simulink model "Boost_Converter_e"  (R2018b)
settings: Solver=VariableStepAuto  StartTime=0.0  StopTime=0.05  RelTol=1e-3
libraries: powerlib x21, pePowerMeasurement x4, powerlib_meascontrol x2
settings Model: Creator=Asus  LastModifiedBy=Asus

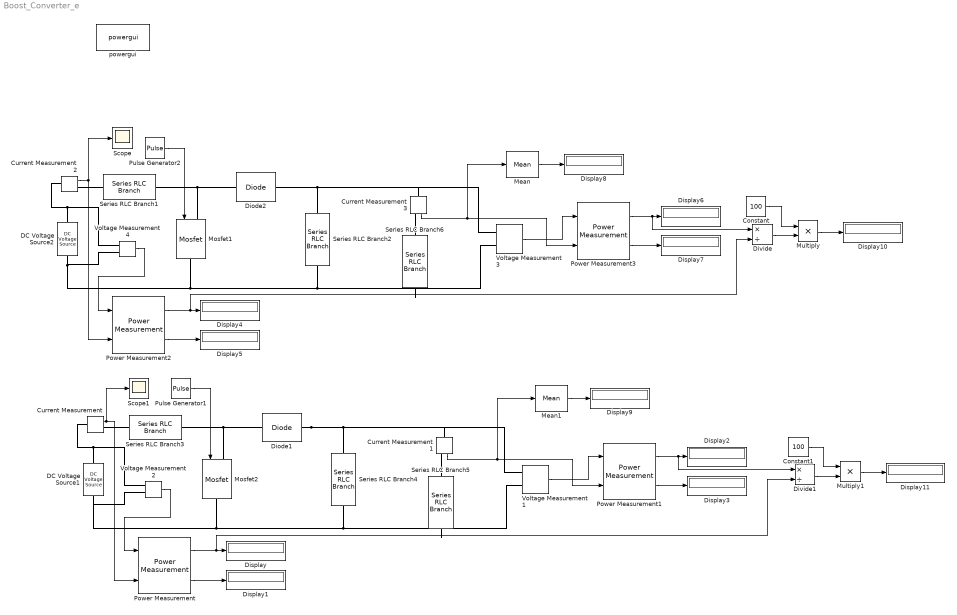
== system Boost_Converter_e ==
  Constant : Constant  Value=100
  Constant1 : Constant  Value=100
  Current Measurement{,1..3} (4 alike) : powerlib/Measurements/Current Measurement  PhasorSimulation=off  OutputType=Complex  PSBequivalent=0
  DC Voltage Source1 : powerlib/Electrical Sources/DC Voltage Source  Amplitude=15  Measurements=None
  DC Voltage Source2 : powerlib/Electrical Sources/DC Voltage Source  Amplitude=15  Measurements=None
  Diode1 : powerlib/Power Electronics/Diode  Ron=0  Lon=0  Vf=0  IC=0  UseSnubber=0  Rs=inf  Cs=inf  Measurements=off
  Diode2 : powerlib/Power Electronics/Diode  Ron=0  Lon=0  Vf=0  IC=0  UseSnubber=0  Rs=inf  Cs=inf  Measurements=off
  Display{,1..11} (12 alike) : Display
  Divide : Product  Inputs=*/
  Divide1 : Product  Inputs=*/
  Mean : powerlib_meascontrol/Measurements/Mean  Freq=500000  Vinit=0  Ts=0
  Mean1 : powerlib_meascontrol/Measurements/Mean  Freq=500000  Vinit=0  Ts=0
  Mosfet1 : powerlib/Power Electronics/Mosfet  Ron=0  Lon=0  Rd=0  Vfd=0  IC=0  Rs=inf  Cs=inf  Measurements=off
  Mosfet2 : powerlib/Power Electronics/Mosfet  Ron=0  Lon=0  Rd=0  Vfd=0  IC=0  Rs=inf  Cs=inf  Measurements=off
  Multiply : Product
  Multiply1 : Product
  Power Measurement{,1..3} (4 alike) : pePowerMeasurement/Power Measurement  LabelModeActiveChoice=Continuous  F=50000  K=[0 1 2 3]  Ts=0
  Pulse Generator1 : DiscretePulseGenerator  PulseType=Time based  Period=1/500000  PulseWidth=37.5
  Pulse Generator2 : DiscretePulseGenerator  PulseType=Time based  Period=1/500000  PulseWidth=37.5
  Scope : Scope
  Scope1 : Scope
  Series RLC Branch1 : powerlib/Elements/Series RLC Branch  LConnTagsString=__new0  RConnTagsString=__new0  BranchType=L  Resistance=57e-3  Inductance=8.53e-6  SetiL0=off  InitialCurrent=0  Capacitance=1e-6  Setx0=off  InitialVoltage=0  Measurements=None
  Series RLC Branch2 : powerlib/Elements/Series RLC Branch  LConnTagsString=__new0  RConnTagsString=__new0  BranchType=C  Resistance=1  Inductance=1e-3  SetiL0=off  InitialCurrent=0  Capacitance=3.125e-6  Setx0=off  InitialVoltage=0  Measurements=None
  Series RLC Branch3 : powerlib/Elements/Series RLC Branch  LConnTagsString=__new0  RConnTagsString=__new0  BranchType=RL  Resistance=57e-3  Inductance=8.53e-6  SetiL0=off  InitialCurrent=0  Capacitance=1e-6  Setx0=off  InitialVoltage=0  Measurements=None
  Series RLC Branch4 : powerlib/Elements/Series RLC Branch  LConnTagsString=__new0  RConnTagsString=__new0  BranchType=C  Resistance=1  Inductance=1e-3  SetiL0=off  InitialCurrent=0  Capacitance=3.125e-6  Setx0=off  InitialVoltage=0  Measurements=None
  Series RLC Branch5 : powerlib/Elements/Series RLC Branch  LConnTagsString=__new0  RConnTagsString=__new0  BranchType=R  Resistance=12  Inductance=1e-3  SetiL0=off  InitialCurrent=0  Capacitance=1e-6  Setx0=off  InitialVoltage=0  Measurements=None
  Series RLC Branch6 : powerlib/Elements/Series RLC Branch  LConnTagsString=__new0  RConnTagsString=__new0  BranchType=R  Resistance=12  Inductance=1e-3  SetiL0=off  InitialCurrent=0  Capacitance=1e-6  Setx0=off  InitialVoltage=0  Measurements=None
  Voltage Measurement{1..4} (4 alike) : powerlib/Measurements/Voltage Measurement  PhasorSimulation=off  OutputType=Complex  PSBequivalent=0
  powergui : powerlib/powergui  Priority=1  SimulationMode=Continuous  SampleTime=50e-6  frequency=60  Iterations=50  frequencyindice=0  Pbase=100e6  ErrMax=1e-4  UnitsV=kV  UnitsW=MW  buscounter=0  FunctionMessages=off  echomessages=off  EnableUseOfTLC=off  CurrentSourceSwitches=off  DisableSnubberDevices=off  DisableRonSwitches=off  DisableVfSwitches=off  DisplayEquations=off  SolverType=Tustin/Backward Euler (TBE)  Interpol=off  ExternalGateDelay=off  methode=off  Ts=100  x0status=blocks  SPID=on  SwTol=0  HookPort=off  RestoreLinks=warning  ResistiveCurrentMeasurement=off  Frange=[0:2:500]  Ylog=off  Xlog=on  ShowGrid=off  save=off  variable=ZData  structure=0  ZoomFFT=off  StartTime=0.0  cycles=1  DisplayStyle=1  fundamental=60  FreqAxis=off  MaxFrequency=1000  frequencyindicesteady=1  RmsSteady=1  display=off
  wires:
  Pulse Generator1/1 -> Mosfet2/1
  Voltage Measurement2/1 -> Power Measurement/1
  Current Measurement/1 -> Scope1/1, Power Measurement/2
  Power Measurement/1 -> Divide1/2, Display/1
  Power Measurement/2 -> Display1/1
  Current Measurement1/1 -> Mean1/1, Power Measurement1/2
  Voltage Measurement1/1 -> Power Measurement1/1
  Power Measurement1/1 -> Divide1/1, Display2/1
  Power Measurement1/2 -> Display3/1
  Voltage Measurement3/1 -> Power Measurement3/1
  Voltage Measurement4/1 -> Power Measurement2/1
  Power Measurement2/1 -> Divide/2, Display4/1
  Power Measurement3/2 -> Display7/1
  Power Measurement2/2 -> Display5/1
  Power Measurement3/1 -> Divide/1, Display6/1
  Current Measurement3/1 -> Mean/1, Power Measurement3/2
  Pulse Generator2/1 -> Mosfet1/1
  Current Measurement2/1 -> Scope/1, Power Measurement2/2
  Mean/1 -> Display8/1
  Mean1/1 -> Display9/1
  Divide/1 -> Multiply/2
  Constant/1 -> Multiply/1
  Multiply/1 -> Display10/1
  Divide1/1 -> Multiply1/2
  Multiply1/1 -> Display11/1
  Constant1/1 -> Multiply1/1
  connections:
  Series RLC Branch4/RConn1 -- Series RLC Branch5/RConn1 -- Voltage Measurement1/LConn2 -- Voltage Measurement2/LConn2 -- DC Voltage Source1/LConn1 -- Mosfet2/RConn1
  Diode1/RConn1 -- Voltage Measurement1/LConn1 -- Current Measurement1/LConn1 -- Series RLC Branch4/LConn1
  Diode1/LConn1 -- Mosfet2/LConn1 -- Series RLC Branch3/RConn1
  Current Measurement/LConn1 -- Voltage Measurement2/LConn1 -- DC Voltage Source1/RConn1
  Current Measurement/RConn1 -- Series RLC Branch3/LConn1
  Current Measurement1/RConn1 -- Series RLC Branch5/LConn1
  DC Voltage Source2/LConn1 -- Series RLC Branch2/RConn1 -- Series RLC Branch6/RConn1 -- Voltage Measurement3/LConn2 -- Mosfet1/RConn1 -- Voltage Measurement4/LConn2
  Series RLC Branch1/RConn1 -- Diode2/LConn1 -- Mosfet1/LConn1
  Current Measurement2/LConn1 -- Voltage Measurement4/LConn1 -- DC Voltage Source2/RConn1
  Series RLC Branch2/LConn1 -- Diode2/RConn1 -- Voltage Measurement3/LConn1 -- Current Measurement3/LConn1
  Current Measurement3/RConn1 -- Series RLC Branch6/LConn1
  Current Measurement2/RConn1 -- Series RLC Branch1/LConn1
